simulink model "VTOL_Simulink"  (R2023a)
settings: Solver=ode4  StartTime=0.0  StopTime=100  FixedStep=0.001  RelTol=1e-3
values from neighbouring files (symbols this model uses):
  C_p = K_T/(0.5*rho*S_p*(R_p)^2)    (= 0.0365795108738)    [vtol_script.m]
  c_w = 0.35    [vtol_script.m]
  CD_0 = 0.028225    [vtol_script.m]
  CL_0 = 0.669072    [vtol_script.m]
  CL_a = 0.0904/D2R    (= 5.17953846798)    [vtol_script.m]
  Cl_beta = del_Cl_beta    (= 0.0002)    [vtol_script.m]
  Cm_0 = 0.051262    [vtol_script.m]
  Cm_a = -0.0144155/D2R    (= -0.825947309571)    [vtol_script.m]
  g = 9.8    [vtol_script.m]
  guidance_mode_on = 1    [vtol_script.m]
  K_motor = 942.3726    [vtol_script.m]
  Kinduce = 1/(pi*e*AR)    (= 0.0461549334966)    [vtol_script.m]
  m_plane = 7    [vtol_script.m]
  q_motor = 283    [vtol_script.m]
  R_p = 0.3556/2    (= 0.1778)    [vtol_script.m]
  S_p = pi*(R_p)^2    (= 0.0993146659031)    [vtol_script.m]
  S_ref = 0.704    [vtol_script.m]
  Wspan = 2.5    [vtol_script.m]
undefined symbols (not defined in the file or in its folder): alpha_thoff, Earth, sigbuilder_block, WGS84
libraries: slpidlib x13, matrix_library x4, simulink_extras x3, sharedtransform x2, aerolibasang x1, aerolibatmos2 x1, aerolibtransform2 x1, shared6dof x1
(part 2 of 2)

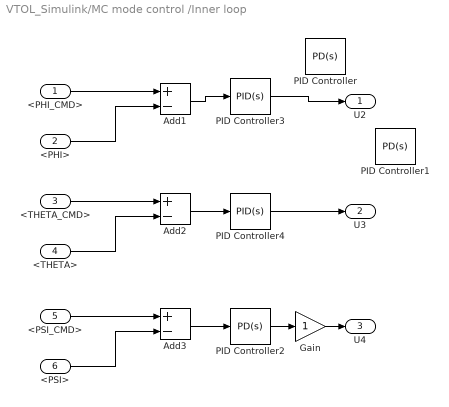
== system VTOL_Simulink/MC mode control /Inner loop ==
  " <PHI_CMD>" : Inport
  <PHI> : Inport  Port=2
  " <THETA_CMD>" : Inport  Port=3
  <THETA> : Inport  Port=4
  <PSI_CMD> : Inport  Port=5
  <PSI> : Inport  Port=6
  Add1 : Sum  Inputs=+-
  Add2 : Sum  Inputs=+-
  Add3 : Sum  Inputs=+-
  Gain : Gain
  PID Controller : slpidlib/PID Controller  Controller=PD  Form=Parallel  TimeDomain=Continuous-time  UseExternalTs=off  SampleTime=-1  IntegratorMethod=Forward Euler  FilterMethod=Forward Euler  ControllerParametersSource=internal  P=5  I=1  UseKiTs=off  D=0.5  N=100  UseFilter=on  TunerSelectOption=Transfer Function Based (PID Tuner App)  InitialConditionSource=internal  InitialConditionForIntegrator=0  InitialConditionForFilter=0  DifferentiatorICPrevScaledInput=0  ExternalReset=none  TrackingMode=off  Kt=1  LimitOutput=off  SatLimitsSource=internal  UpperSaturationLimit=inf  LowerSaturationLimit=-inf  LinearizeAsGain=on  AntiWindupMode=none  Kb=1  LimitIntegrator=off  UpperIntegratorSaturationLimit=inf  LowerIntegratorSaturationLimit=-inf  POutMin=[]  POutMax=[]  IOutMin=[]  IOutMax=[]  DOutMin=[]  DOutMax=[]  NOutMin=[]  NOutMax=[]  SumOutMin=[]  SumOutMax=[]  SaturationOutMin=[]  SaturationOutMax=[]  PParamMin=[]  PParamMax=[]  IParamMin=[]  IParamMax=[]  DParamMin=[]  DParamMax=[]  NParamMin=[]  NParamMax=[]  KbParamMin=[]  KbParamMax=[]  KtParamMin=[]  KtParamMax=[]  KbOutMin=[]  KbOutMax=[]  KtOutMin=[]  KtOutMax=[]  IntegratorOutMin=[]  IntegratorOutMax=[]  FilterOutMin=[]  FilterOutMax=[]  SumI1OutMin=[]  SumI1OutMax=[]  SumI2OutMin=[]  SumI2OutMax=[]  SumI3OutMin=[]  SumI3OutMax=[]  SumI4OutMin=[]  SumI4OutMax=[]  SumDOutMin=[]  SumDOutMax=[]  DifferentiatorOutMin=[]  DifferentiatorOutMax=[]  FilterDiffOutCoefMin=[]  FilterDiffOutCoefMax=[]  ReciprocalOutMin=[]  ReciprocalOutMax=[]  SumDenOutMin=[]  SumDenOutMax=[]  SumNumOutMin=[]  SumNumOutMax=[]  DivideOutMin=[]  DivideOutMax=[]  UdiffTsProdOutMin=[]  UdiffTsProdOutMax=[]  NTsProdOutMin=[]  NTsProdOutMax=[]  UintegralTsProdOutMin=[]  UintegralTsProdOutMax=[]  UngainTsProdOutMin=[]  UngainTsProdOutMax=[]  ClampingZeroOutDataTypeStr=Inherit: Inherit via back propagation  ClampingZeroOutMin=[]  ClampingZeroOutMax=[]  FilterDenConstantOutDataTypeStr=Inherit: Inherit via back propagation  FilterDenConstantOutMin=[]  FilterDenConstantOutMax=[]  PCopyOutDataTypeStr=Inherit: Inherit via back propagation  PCopyOutMin=[]  PCopyOutMax=[]  NCopyOutDataTypeStr=Inherit: Inherit via back propagation  NCopyOutMin=[]  NCopyOutMax=[]  IntegratorContinuousStateAttributes=''  IntegratorStateMustResolveToSignalObject=off  IntegratorRTWStateStorageClass=Auto  FilterContinuousStateAttributes=''  FilterStateMustResolveToSignalObject=off  FilterRTWStateStorageClass=Auto  ParallelPVariant=InternalParameters  IdealPVariant=Disabled  IVariant=Disabled  DVariant=InternalParameters  IntegratorVariant=Disabled  SatVariant=Disabled  AWVariant=Disabled  PCopyVariant=Disabled  TRVariant=Disabled  FdbkBlocksVariant=Forward  IdealPFdbkVariant=Disabled  SatFdbkVariant=Disabled  DerivativeFilterVariant=ContFilter  NVariant=InternalParameters  NCopyVariant=Disabled  FilterICVariant=InternalICsFilter  IntegratorICVariant=Disabled  ExternalResetVariant=Disabled  TRSumVariant=Passthrough  SumFdbkVariant=Disabled  SumVariant=Sum_PD  TsampFilterVariant=InternalTs  TsampNgainVariant=Passthrough  TsampIntegralVariant=Disabled_SignalSpec  ExternalSaturationOutDataTypeStr=Inherit: Same as second input
  PID Controller1 : slpidlib/PID Controller  Controller=PD  Form=Parallel  TimeDomain=Continuous-time  UseExternalTs=off  SampleTime=-1  IntegratorMethod=Forward Euler  FilterMethod=Forward Euler  ControllerParametersSource=internal  P=5  I=1  UseKiTs=off  D=0.5  N=100  UseFilter=on  TunerSelectOption=Transfer Function Based (PID Tuner App)  InitialConditionSource=internal  InitialConditionForIntegrator=0  InitialConditionForFilter=0  DifferentiatorICPrevScaledInput=0  ExternalReset=none  TrackingMode=off  Kt=1  LimitOutput=off  SatLimitsSource=internal  UpperSaturationLimit=inf  LowerSaturationLimit=-inf  LinearizeAsGain=on  AntiWindupMode=none  Kb=1  LimitIntegrator=off  UpperIntegratorSaturationLimit=inf  LowerIntegratorSaturationLimit=-inf  POutMin=[]  POutMax=[]  IOutMin=[]  IOutMax=[]  DOutMin=[]  DOutMax=[]  NOutMin=[]  NOutMax=[]  SumOutMin=[]  SumOutMax=[]  SaturationOutMin=[]  SaturationOutMax=[]  PParamMin=[]  PParamMax=[]  IParamMin=[]  IParamMax=[]  DParamMin=[]  DParamMax=[]  NParamMin=[]  NParamMax=[]  KbParamMin=[]  KbParamMax=[]  KtParamMin=[]  KtParamMax=[]  KbOutMin=[]  KbOutMax=[]  KtOutMin=[]  KtOutMax=[]  IntegratorOutMin=[]  IntegratorOutMax=[]  FilterOutMin=[]  FilterOutMax=[]  SumI1OutMin=[]  SumI1OutMax=[]  SumI2OutMin=[]  SumI2OutMax=[]  SumI3OutMin=[]  SumI3OutMax=[]  SumI4OutMin=[]  SumI4OutMax=[]  SumDOutMin=[]  SumDOutMax=[]  DifferentiatorOutMin=[]  DifferentiatorOutMax=[]  FilterDiffOutCoefMin=[]  FilterDiffOutCoefMax=[]  ReciprocalOutMin=[]  ReciprocalOutMax=[]  SumDenOutMin=[]  SumDenOutMax=[]  SumNumOutMin=[]  SumNumOutMax=[]  DivideOutMin=[]  DivideOutMax=[]  UdiffTsProdOutMin=[]  UdiffTsProdOutMax=[]  NTsProdOutMin=[]  NTsProdOutMax=[]  UintegralTsProdOutMin=[]  UintegralTsProdOutMax=[]  UngainTsProdOutMin=[]  UngainTsProdOutMax=[]  ClampingZeroOutDataTypeStr=Inherit: Inherit via back propagation  ClampingZeroOutMin=[]  ClampingZeroOutMax=[]  FilterDenConstantOutDataTypeStr=Inherit: Inherit via back propagation  FilterDenConstantOutMin=[]  FilterDenConstantOutMax=[]  PCopyOutDataTypeStr=Inherit: Inherit via back propagation  PCopyOutMin=[]  PCopyOutMax=[]  NCopyOutDataTypeStr=Inherit: Inherit via back propagation  NCopyOutMin=[]  NCopyOutMax=[]  IntegratorContinuousStateAttributes=''  IntegratorStateMustResolveToSignalObject=off  IntegratorRTWStateStorageClass=Auto  FilterContinuousStateAttributes=''  FilterStateMustResolveToSignalObject=off  FilterRTWStateStorageClass=Auto  ParallelPVariant=InternalParameters  IdealPVariant=Disabled  IVariant=Disabled  DVariant=InternalParameters  IntegratorVariant=Disabled  SatVariant=Disabled  AWVariant=Disabled  PCopyVariant=Disabled  TRVariant=Disabled  FdbkBlocksVariant=Forward  IdealPFdbkVariant=Disabled  SatFdbkVariant=Disabled  DerivativeFilterVariant=ContFilter  NVariant=InternalParameters  NCopyVariant=Disabled  FilterICVariant=InternalICsFilter  IntegratorICVariant=Disabled  ExternalResetVariant=Disabled  TRSumVariant=Passthrough  SumFdbkVariant=Disabled  SumVariant=Sum_PD  TsampFilterVariant=InternalTs  TsampNgainVariant=Passthrough  TsampIntegralVariant=Disabled_SignalSpec  ExternalSaturationOutDataTypeStr=Inherit: Same as second input
  PID Controller2 : slpidlib/PID Controller  Controller=PD  Form=Parallel  TimeDomain=Continuous-time  UseExternalTs=off  SampleTime=-1  IntegratorMethod=Forward Euler  FilterMethod=Forward Euler  ControllerParametersSource=internal  P=1  I=1  UseKiTs=off  D=0  N=100  UseFilter=on  TunerSelectOption=Transfer Function Based (PID Tuner App)  InitialConditionSource=internal  InitialConditionForIntegrator=0  InitialConditionForFilter=0  DifferentiatorICPrevScaledInput=0  ExternalReset=none  TrackingMode=off  Kt=1  LimitOutput=off  SatLimitsSource=internal  UpperSaturationLimit=inf  LowerSaturationLimit=-inf  LinearizeAsGain=on  AntiWindupMode=none  Kb=1  LimitIntegrator=off  UpperIntegratorSaturationLimit=inf  LowerIntegratorSaturationLimit=-inf  POutMin=[]  POutMax=[]  IOutMin=[]  IOutMax=[]  DOutMin=[]  DOutMax=[]  NOutMin=[]  NOutMax=[]  SumOutMin=[]  SumOutMax=[]  SaturationOutMin=[]  SaturationOutMax=[]  PParamMin=[]  PParamMax=[]  IParamMin=[]  IParamMax=[]  DParamMin=[]  DParamMax=[]  NParamMin=[]  NParamMax=[]  KbParamMin=[]  KbParamMax=[]  KtParamMin=[]  KtParamMax=[]  KbOutMin=[]  KbOutMax=[]  KtOutMin=[]  KtOutMax=[]  IntegratorOutMin=[]  IntegratorOutMax=[]  FilterOutMin=[]  FilterOutMax=[]  SumI1OutMin=[]  SumI1OutMax=[]  SumI2OutMin=[]  SumI2OutMax=[]  SumI3OutMin=[]  SumI3OutMax=[]  SumI4OutMin=[]  SumI4OutMax=[]  SumDOutMin=[]  SumDOutMax=[]  DifferentiatorOutMin=[]  DifferentiatorOutMax=[]  FilterDiffOutCoefMin=[]  FilterDiffOutCoefMax=[]  ReciprocalOutMin=[]  ReciprocalOutMax=[]  SumDenOutMin=[]  SumDenOutMax=[]  SumNumOutMin=[]  SumNumOutMax=[]  DivideOutMin=[]  DivideOutMax=[]  UdiffTsProdOutMin=[]  UdiffTsProdOutMax=[]  NTsProdOutMin=[]  NTsProdOutMax=[]  UintegralTsProdOutMin=[]  UintegralTsProdOutMax=[]  UngainTsProdOutMin=[]  UngainTsProdOutMax=[]  ClampingZeroOutDataTypeStr=Inherit: Inherit via back propagation  ClampingZeroOutMin=[]  ClampingZeroOutMax=[]  FilterDenConstantOutDataTypeStr=Inherit: Inherit via back propagation  FilterDenConstantOutMin=[]  FilterDenConstantOutMax=[]  PCopyOutDataTypeStr=Inherit: Inherit via back propagation  PCopyOutMin=[]  PCopyOutMax=[]  NCopyOutDataTypeStr=Inherit: Inherit via back propagation  NCopyOutMin=[]  NCopyOutMax=[]  IntegratorContinuousStateAttributes=''  IntegratorStateMustResolveToSignalObject=off  IntegratorRTWStateStorageClass=Auto  FilterContinuousStateAttributes=''  FilterStateMustResolveToSignalObject=off  FilterRTWStateStorageClass=Auto  ParallelPVariant=InternalParameters  IdealPVariant=Disabled  IVariant=Disabled  DVariant=InternalParameters  IntegratorVariant=Disabled  SatVariant=Disabled  AWVariant=Disabled  PCopyVariant=Disabled  TRVariant=Disabled  FdbkBlocksVariant=Forward  IdealPFdbkVariant=Disabled  SatFdbkVariant=Disabled  DerivativeFilterVariant=ContFilter  NVariant=InternalParameters  NCopyVariant=Disabled  FilterICVariant=InternalICsFilter  IntegratorICVariant=Disabled  ExternalResetVariant=Disabled  TRSumVariant=Passthrough  SumFdbkVariant=Disabled  SumVariant=Sum_PD  TsampFilterVariant=InternalTs  TsampNgainVariant=Passthrough  TsampIntegralVariant=Disabled_SignalSpec  ExternalSaturationOutDataTypeStr=Inherit: Same as second input
  PID Controller3 : slpidlib/PID Controller  Controller=PID  Form=Parallel  TimeDomain=Continuous-time  UseExternalTs=off  SampleTime=-1  IntegratorMethod=Forward Euler  FilterMethod=Forward Euler  ControllerParametersSource=internal  P=25  I=0.01  UseKiTs=off  D=0.01  N=100  UseFilter=on  TunerSelectOption=Transfer Function Based (PID Tuner App)  InitialConditionSource=internal  InitialConditionForIntegrator=0  InitialConditionForFilter=0  DifferentiatorICPrevScaledInput=0  ExternalReset=none  TrackingMode=off  Kt=1  LimitOutput=off  SatLimitsSource=internal  UpperSaturationLimit=inf  LowerSaturationLimit=-inf  LinearizeAsGain=on  AntiWindupMode=none  Kb=1  LimitIntegrator=off  UpperIntegratorSaturationLimit=inf  LowerIntegratorSaturationLimit=-inf  POutMin=[]  POutMax=[]  IOutMin=[]  IOutMax=[]  DOutMin=[]  DOutMax=[]  NOutMin=[]  NOutMax=[]  SumOutMin=[]  SumOutMax=[]  SaturationOutMin=[]  SaturationOutMax=[]  PParamMin=[]  PParamMax=[]  IParamMin=[]  IParamMax=[]  DParamMin=[]  DParamMax=[]  NParamMin=[]  NParamMax=[]  KbParamMin=[]  KbParamMax=[]  KtParamMin=[]  KtParamMax=[]  KbOutMin=[]  KbOutMax=[]  KtOutMin=[]  KtOutMax=[]  IntegratorOutMin=[]  IntegratorOutMax=[]  FilterOutMin=[]  FilterOutMax=[]  SumI1OutMin=[]  SumI1OutMax=[]  SumI2OutMin=[]  SumI2OutMax=[]  SumI3OutMin=[]  SumI3OutMax=[]  SumI4OutMin=[]  SumI4OutMax=[]  SumDOutMin=[]  SumDOutMax=[]  DifferentiatorOutMin=[]  DifferentiatorOutMax=[]  FilterDiffOutCoefMin=[]  FilterDiffOutCoefMax=[]  ReciprocalOutMin=[]  ReciprocalOutMax=[]  SumDenOutMin=[]  SumDenOutMax=[]  SumNumOutMin=[]  SumNumOutMax=[]  DivideOutMin=[]  DivideOutMax=[]  UdiffTsProdOutMin=[]  UdiffTsProdOutMax=[]  NTsProdOutMin=[]  NTsProdOutMax=[]  UintegralTsProdOutMin=[]  UintegralTsProdOutMax=[]  UngainTsProdOutMin=[]  UngainTsProdOutMax=[]  ClampingZeroOutDataTypeStr=Inherit: Inherit via back propagation  ClampingZeroOutMin=[]  ClampingZeroOutMax=[]  FilterDenConstantOutDataTypeStr=Inherit: Inherit via back propagation  FilterDenConstantOutMin=[]  FilterDenConstantOutMax=[]  PCopyOutDataTypeStr=Inherit: Inherit via back propagation  PCopyOutMin=[]  PCopyOutMax=[]  NCopyOutDataTypeStr=Inherit: Inherit via back propagation  NCopyOutMin=[]  NCopyOutMax=[]  IntegratorContinuousStateAttributes=''  IntegratorStateMustResolveToSignalObject=off  IntegratorRTWStateStorageClass=Auto  FilterContinuousStateAttributes=''  FilterStateMustResolveToSignalObject=off  FilterRTWStateStorageClass=Auto  ParallelPVariant=InternalParameters  IdealPVariant=Disabled  IVariant=InternalParameters  DVariant=InternalParameters  IntegratorVariant=Continuous  SatVariant=Disabled  AWVariant=Passthrough  PCopyVariant=Disabled  TRVariant=Disabled  FdbkBlocksVariant=Forward  IdealPFdbkVariant=Disabled  SatFdbkVariant=Disabled  DerivativeFilterVariant=ContFilter  NVariant=InternalParameters  NCopyVariant=Disabled  FilterICVariant=InternalICsFilter  IntegratorICVariant=InternalICs  ExternalResetVariant=Disabled  TRSumVariant=Passthrough  SumFdbkVariant=Disabled  SumVariant=Sum_PID  TsampFilterVariant=InternalTs  TsampNgainVariant=Passthrough  TsampIntegralVariant=Disabled_SignalSpec  ExternalSaturationOutDataTypeStr=Inherit: Same as second input
  PID Controller4 : slpidlib/PID Controller  Controller=PID  Form=Parallel  TimeDomain=Continuous-time  UseExternalTs=off  SampleTime=-1  IntegratorMethod=Forward Euler  FilterMethod=Forward Euler  ControllerParametersSource=internal  P=30  I=0.01  UseKiTs=off  D=0.01  N=100  UseFilter=on  TunerSelectOption=Transfer Function Based (PID Tuner App)  InitialConditionSource=internal  InitialConditionForIntegrator=0  InitialConditionForFilter=0  DifferentiatorICPrevScaledInput=0  ExternalReset=none  TrackingMode=off  Kt=1  LimitOutput=off  SatLimitsSource=internal  UpperSaturationLimit=inf  LowerSaturationLimit=-inf  LinearizeAsGain=on  AntiWindupMode=none  Kb=1  LimitIntegrator=off  UpperIntegratorSaturationLimit=inf  LowerIntegratorSaturationLimit=-inf  POutMin=[]  POutMax=[]  IOutMin=[]  IOutMax=[]  DOutMin=[]  DOutMax=[]  NOutMin=[]  NOutMax=[]  SumOutMin=[]  SumOutMax=[]  SaturationOutMin=[]  SaturationOutMax=[]  PParamMin=[]  PParamMax=[]  IParamMin=[]  IParamMax=[]  DParamMin=[]  DParamMax=[]  NParamMin=[]  NParamMax=[]  KbParamMin=[]  KbParamMax=[]  KtParamMin=[]  KtParamMax=[]  KbOutMin=[]  KbOutMax=[]  KtOutMin=[]  KtOutMax=[]  IntegratorOutMin=[]  IntegratorOutMax=[]  FilterOutMin=[]  FilterOutMax=[]  SumI1OutMin=[]  SumI1OutMax=[]  SumI2OutMin=[]  SumI2OutMax=[]  SumI3OutMin=[]  SumI3OutMax=[]  SumI4OutMin=[]  SumI4OutMax=[]  SumDOutMin=[]  SumDOutMax=[]  DifferentiatorOutMin=[]  DifferentiatorOutMax=[]  FilterDiffOutCoefMin=[]  FilterDiffOutCoefMax=[]  ReciprocalOutMin=[]  ReciprocalOutMax=[]  SumDenOutMin=[]  SumDenOutMax=[]  SumNumOutMin=[]  SumNumOutMax=[]  DivideOutMin=[]  DivideOutMax=[]  UdiffTsProdOutMin=[]  UdiffTsProdOutMax=[]  NTsProdOutMin=[]  NTsProdOutMax=[]  UintegralTsProdOutMin=[]  UintegralTsProdOutMax=[]  UngainTsProdOutMin=[]  UngainTsProdOutMax=[]  ClampingZeroOutDataTypeStr=Inherit: Inherit via back propagation  ClampingZeroOutMin=[]  ClampingZeroOutMax=[]  FilterDenConstantOutDataTypeStr=Inherit: Inherit via back propagation  FilterDenConstantOutMin=[]  FilterDenConstantOutMax=[]  PCopyOutDataTypeStr=Inherit: Inherit via back propagation  PCopyOutMin=[]  PCopyOutMax=[]  NCopyOutDataTypeStr=Inherit: Inherit via back propagation  NCopyOutMin=[]  NCopyOutMax=[]  IntegratorContinuousStateAttributes=''  IntegratorStateMustResolveToSignalObject=off  IntegratorRTWStateStorageClass=Auto  FilterContinuousStateAttributes=''  FilterStateMustResolveToSignalObject=off  FilterRTWStateStorageClass=Auto  ParallelPVariant=InternalParameters  IdealPVariant=Disabled  IVariant=InternalParameters  DVariant=InternalParameters  IntegratorVariant=Continuous  SatVariant=Disabled  AWVariant=Passthrough  PCopyVariant=Disabled  TRVariant=Disabled  FdbkBlocksVariant=Forward  IdealPFdbkVariant=Disabled  SatFdbkVariant=Disabled  DerivativeFilterVariant=ContFilter  NVariant=InternalParameters  NCopyVariant=Disabled  FilterICVariant=InternalICsFilter  IntegratorICVariant=InternalICs  ExternalResetVariant=Disabled  TRSumVariant=Passthrough  SumFdbkVariant=Disabled  SumVariant=Sum_PID  TsampFilterVariant=InternalTs  TsampNgainVariant=Passthrough  TsampIntegralVariant=Disabled_SignalSpec  ExternalSaturationOutDataTypeStr=Inherit: Same as second input
  " U2" : Outport
  U3 : Outport  Port=2
  U4 : Outport  Port=3
  wires:
  <PHI>/1 -> Add1/2
  <THETA>/1 -> Add2/2
  <PSI>/1 -> Add3/2
  Add1/1 -> PID Controller3/1
  Add2/1 -> PID Controller4/1
  Add3/1 -> PID Controller2/1
  PID Controller3/1 -> " U2"/1
  PID Controller4/1 -> U3/1
  PID Controller2/1 -> Gain/1
  <PSI_CMD>/1 -> Add3/1
  Gain/1 -> U4/1
  " <PHI_CMD>"/1 -> Add1/1
  " <THETA_CMD>"/1 -> Add2/1

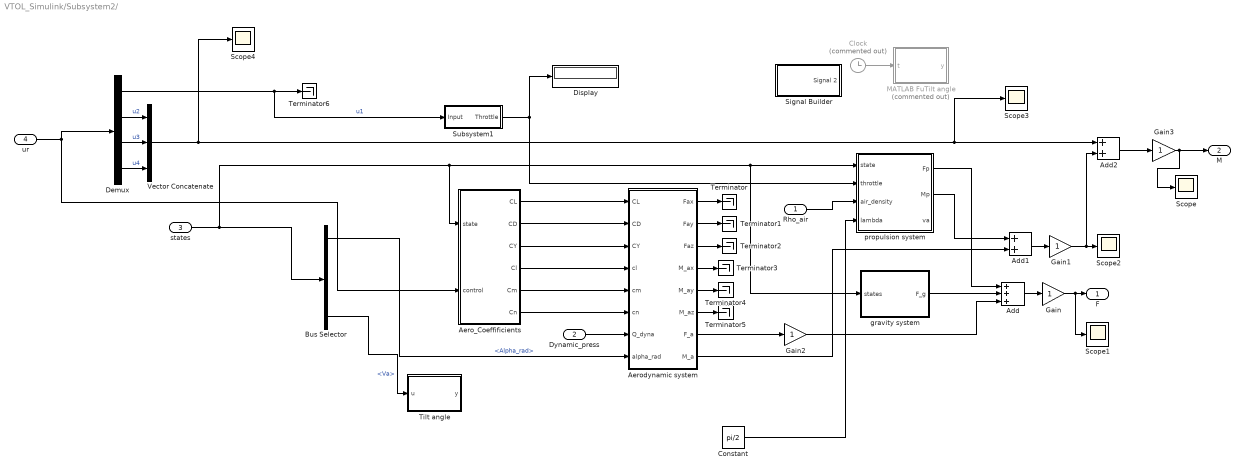
== system VTOL_Simulink/Subsystem2/  ==
  " Rho_air" : Inport
  Dynamic_press : Inport  Port=2
  states : Inport  Port=3
  ur : Inport  Port=4
  " Aero_Coeffificients" : Subsystem
  " gravity system" : Subsystem
  " propulsion system" : Subsystem
  Add : Sum  Inputs=+++
  Add1 : Sum
  Add2 : Sum
  Aerodynamic system : Subsystem
  Bus Selector : BusSelector  OutputSignals=Alpha_rad,pn pe pd,Euler_ang_rad,Va
  Clock : Clock  Commented=on
  Constant : Constant  Value=pi/2
  Demux : Demux  Outputs=04
  Display : Display
  Gain{,1..3} (4 alike) : Gain
  MATLAB FuTilt angle : MATLAB Function  Commented=on  TreatAsAtomicUnit=on
  Scope{,1..4} (5 alike) : Scope
  Signal Builder : Subsystem  Tag=STV Subsys  LoadFcn=sigbuilder_block('load');  StartFcn=sigbuilder_block('start');  StopFcn=sigbuilder_block('stop');  ClipboardFcn=sigbuilder_block('clipboard');  mask(Sigbuilder block){tuvar=[0:10]}
      mask help: Simulink:masks:SigbuilderBlock_MD
      mask init:
      | if ~strcmp(get_param(bdroot(gcbh),'SimulationStatus'),'stopped') tuvar = sigbuilder_block('maskInit'); end
      settings: CopyFcn=sigbuilder_block('copy');  DeleteFcn=sigbuilder_block('delete');  ModelCloseFcn=sigbuilder_block('modelClose');  PreSaveFcn=sigbuilder_block('preSave');  PauseFcn=sigbuilder_block('pause');  ContinueFcn=sigbuilder_block('continue');  NameChangeFcn=sigbuilder_block('namechange');  OpenFcn=sigbuilder_block('open',[5.4 36 1141.2 516.6 ]);  CloseFcn=sigbuilder_block('close');
      mask Display: plot(0, 0, 100, 100,[2, 2, 32, 32, 2], [68, 8, 8, 68, 68],[32, 2], [38, 38], [32, 19, 2],[53, 60, 44], [32, 17, 17, 2],[16, 16, 31, 31]);txt = getActiveGroup(gcbh);text(2, 100, txt,'verticalAlignment', 'top');
  Subsystem1 : Subsystem
  Terminator{,1..6} (7 alike) : Terminator
  Tilt angle : MATLAB Function  TreatAsAtomicUnit=on
  Vector Concatenate : Concatenate  NumInputs=03
  F : Outport
  " M" : Outport  Port=2
  wires:
  Aerodynamic system/4(" M_ax") -> Terminator3/1
  " Aero_Coeffificients"/4("  Cl") -> Aerodynamic system/4(" cl")
  " Aero_Coeffificients"/5("  Cm") -> Aerodynamic system/5(" cm")
  Aerodynamic system/5(M_ay) -> Terminator4/1
  Aerodynamic system/2(" Fay") -> Terminator1/1
  Add/1 -> Gain/1
  Aerodynamic system/3(" Faz") -> Terminator2/1
  " Aero_Coeffificients"/6(" Cn") -> Aerodynamic system/6(" cn")
  " Aero_Coeffificients"/1(" CL") -> Aerodynamic system/1(CL)
  Aerodynamic system/1(" Fax") -> Terminator/1
  Aerodynamic system/6(" M_az") -> Terminator5/1
  " Aero_Coeffificients"/2(" CD") -> Aerodynamic system/2(CD)
  " Aero_Coeffificients"/3(" CY") -> Aerodynamic system/3(CY)
  Dynamic_press/1 -> Aerodynamic system/7(" Q_dyna")
  Bus Selector/1 -> Aerodynamic system/8("  alpha_rad")  "<Alpha_rad>"
  " Rho_air"/1 -> " propulsion system"/3(" air_density")
  Aerodynamic system/7(" F_a") -> Gain2/1
  Aerodynamic system/8(" M_a") -> Add1/2
  " propulsion system"/2(" Mp") -> Add1/1
  Add1/1 -> Gain1/1
  states/1 -> Bus Selector/1, " Aero_Coeffificients"/1(" state"), " gravity system"/1(states), " propulsion system"/1(" state")
  Gain/1 -> Scope1/1, F/1
  Gain2/1 -> Add/3
  Clock/1 -> MATLAB FuTilt angle/1(t)
  Subsystem1/1(" Throttle") -> Display/1, " propulsion system"/2(" throttle")
  " propulsion system"/1(" Fp") -> Add/1
  " gravity system"/1(F_g) -> Add/2
  ur/1 -> " Aero_Coeffificients"/2(" control"), Demux/1
  Demux/1 -> Subsystem1/1(Input), Terminator6/1  "u1"
  Bus Selector/4 -> Tilt angle/1(u)  "<Va>"
  Vector Concatenate/1 -> Scope4/1, Scope3/1, Add2/1
  Demux/2 -> Vector Concatenate/1  "u2"
  Demux/3 -> Vector Concatenate/2  "u3"
  Demux/4 -> Vector Concatenate/3  "u4"
  Add2/1 -> Gain3/1
  Gain1/1 -> Add2/2, Scope2/1
  Gain3/1 -> Scope/1, " M"/1
  Constant/1 -> " propulsion system"/4(" lambda")

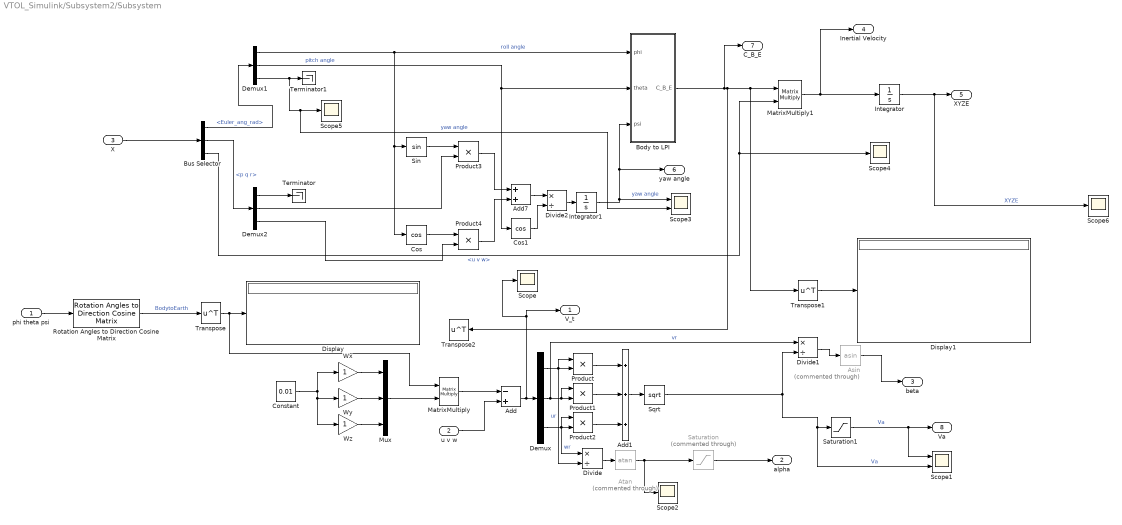
== system VTOL_Simulink/Subsystem2/Subsystem ==
  " phi theta psi" : Inport
  " u v w" : Inport  Port=2
  " X" : Inport  Port=3
  " Body to LPI" : Subsystem
  " Wx" : Gain
  Add : Sum  Inputs=-+
  Add1 : Sum  Inputs=+++
  Add7 : Sum
  Asin : Trigonometry  Commented=through  Operator=asin
  Atan : Trigonometry  Commented=through  Operator=atan
  Bus Selector : BusSelector  OutputSignals=Euler_ang_rad,p q r,u v w
  Constant : Constant  Value=0.01
  Cos : Trigonometry  Operator=cos
  Cos1 : Trigonometry  Operator=cos
  Demux : Demux  Outputs=03
  Demux1 : Demux  Outputs=03
  Demux2 : Demux  Outputs=03
  Display : Display
  Display1 : Display
  Divide : Product  Inputs=*/
  Divide1 : Product  Inputs=*/
  Divide2 : Product  Inputs=*/
  Integrator : Integrator
  Integrator1 : Integrator
  MatrixMultiply : Product  Multiplication=Matrix(*)
  MatrixMultiply1 : Product  Multiplication=Matrix(*)
  Mux : Mux  Inputs=03
  Product{,1..4} (5 alike) : Product
  Rotation Angles to Direction Cosine Matrix : sharedtransform/Rotation Angles to Direction Cosine Matrix  rotationOrder=ZYX  aMode=aMode
  Saturation : Saturate  Commented=through  UpperLimit=pi/6  LowerLimit=-pi/6
  Saturation1 : Saturate  UpperLimit=25  LowerLimit=0
  Scope{,2,4..6} (5 alike) : Scope
  Scope1 : Scope  NumInputPorts=2
  Scope3 : Scope  NumInputPorts=2
  Sin : Trigonometry
  Sqrt : Sqrt
  Terminator : Terminator
  Terminator1 : Terminator
  Transpose : Math  Operator=transpose
  Transpose1 : Math  Operator=transpose
  Transpose2 : Math  Operator=transpose
  Wy : Gain
  Wz : Gain
  " V_t" : Outport
  " alpha" : Outport  Port=2
  " beta" : Outport  Port=3
  " Inertial Velocity " : Outport  Port=4
  XYZE : Outport  Port=5
  yaw angle : Outport  Port=6
  C_B_E : Outport  Port=7
  Va : Outport  Port=8
  wires:
  " u v w"/1 -> Add/2
  " phi theta psi"/1 -> Rotation Angles to Direction Cosine Matrix/1
  Rotation Angles to Direction Cosine Matrix/1 -> Transpose/1  "BodytoEarth"
  Constant/1 -> Wz/1, Wy/1, " Wx"/1
  " Wx"/1 -> Mux/1
  Wy/1 -> Mux/2
  Wz/1 -> Mux/3
  Mux/1 -> MatrixMultiply/2
  MatrixMultiply/1 -> Add/1
  Add/1 -> Scope/1, " V_t"/1, Demux/1
  Demux/1 -> Product/2, Divide/2, Product/1  "ur"
  Demux/2 -> Product1/1, Product1/2, Divide1/1  "vr"
  Demux/3 -> Divide/1, Product2/1, Product2/2  "wr"
  Product/1 -> Add1/1
  Product1/1 -> Add1/2
  Product2/1 -> Add1/3
  Add1/1 -> Sqrt/1
  Sqrt/1 -> Scope1/2, Saturation1/1, Divide1/2  "Va"
  Divide/1 -> Atan/1
  Divide1/1 -> Asin/1
  Atan/1 -> Scope2/1, Saturation/1
  Asin/1 -> " beta"/1
  Cos/1 -> Product4/1
  Demux2/3 -> Product4/2
  Demux1/3 -> Scope3/2, Scope5/1, Terminator1/1  "yaw angle"
  Demux1/2 -> Cos1/1, " Body to LPI"/2(theta)  "pitch angle"
  Demux2/1 -> Terminator/1
  Cos1/1 -> Divide2/2
  Divide2/1 -> Integrator1/1
  Add7/1 -> Divide2/1
  MatrixMultiply1/1 -> Integrator/1, " Inertial Velocity "/1
  Product4/1 -> Add7/2
  Integrator1/1 -> Scope3/1, " Body to LPI"/3(psi), yaw angle/1  "yaw angle"
  Sin/1 -> Product3/1
  Demux2/2 -> Product3/2
  Integrator/1 -> Scope6/1, XYZE/1  "XYZE"
  Product3/1 -> Add7/1
  Demux1/1 -> Cos/1, Sin/1, " Body to LPI"/1(phi)  "roll angle"
  " X"/1 -> Bus Selector/1
  Bus Selector/1 -> Demux1/1  "<Euler_ang_rad>"
  Bus Selector/2 -> Demux2/1  "<p q r>"
  Bus Selector/3 -> MatrixMultiply1/2, Scope4/1  "<u v w>"
  " Body to LPI"/1(C_B_E) -> C_B_E/1, Transpose2/1, Transpose1/1, MatrixMultiply1/1
  Transpose/1 -> MatrixMultiply/1, Display/1
  Transpose1/1 -> Display1/1
  Saturation/1 -> " alpha"/1
  Saturation1/1 -> Scope1/1, Va/1  "Va"

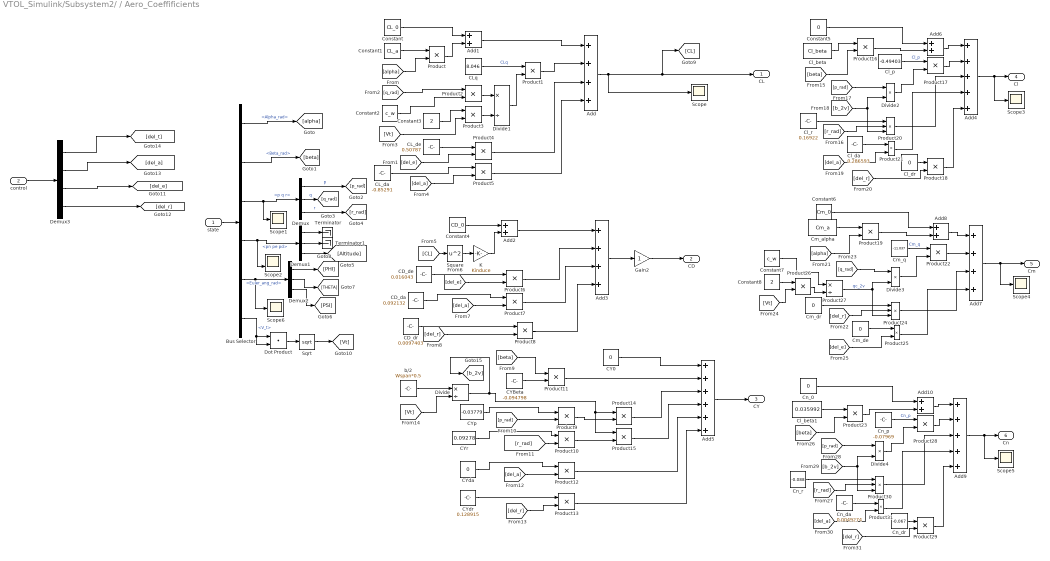
== system VTOL_Simulink/Subsystem2/ / Aero_Coeffificients ==
  " state" : Inport
  " control" : Inport  Port=2
  " CD_da" : Constant  Value=0.092132
  " CD_de" : Constant  Value=0.016043
  " CD_dr" : Constant  Value=0.0097403
  " CL_da" : Constant  Value=-0.85291
  " CL_de" : Constant  Value=0.50787
  " CLq" : Constant  Value=8.046
  " CY0" : Constant  Value=0
  " CYda" : Constant  Value=0
  " CYdr" : Constant  Value=0.128915
  " CYp" : Constant  Value=-0.03779
  " CYr" : Constant  Value=0.09278
  " Cl_beta" : Constant  Value=Cl_beta
  " Cl_beta1" : Constant  Value=0.035992
  " Cl_da" : Constant  Value=0.286593
  " Cl_dr" : Constant  Value=0
  " Cl_p" : Constant  Value=-0.49403
  " Cl_r" : Constant  Value=0.16922
  " Cm_alpha" : Constant  Value=Cm_a
  " Cm_de" : Constant  Value=0
  " Cm_dr" : Constant  Value=0
  " Cm_q" : Constant  Value=-11.037
  " Cn_0" : Constant  Value=0
  " Cn_da" : Constant  Value=0.0049274
  " Cn_dr" : Constant  Value=-0.067
  " Cn_p" : Constant  Value=-0.07969
  " Cn_r" : Constant  Value=-0.088
  " b/2" : Constant  Value=Wspan*0.5
  Add : Sum  Inputs=++++
  Add{1..2,6,8,10} (5 alike) : Sum
  Add3 : Sum  Inputs=++++
  Add4 : Sum  Inputs=+++++
  Add5 : Sum  Inputs=++++++
  Add7 : Sum  Inputs=++++
  Add9 : Sum  Inputs=+++++
  Bus Selector : BusSelector  OutputSignals=Alpha_rad,Beta_rad,p q r,pn pe pd,Euler_ang_rad,V_t
  CYBeta : Constant  Value=-0.094798
  Constant : Constant  Value=CL_0
  Constant1 : Constant  Value=CL_a
  Constant2 : Constant  Value=c_w
  Constant3 : Constant  Value=2
  Constant4 : Constant  Value=CD_0
  Constant5 : Constant  Value=0
  Constant6 : Constant  Value=Cm_0
  Constant7 : Constant  Value=c_w
  Constant8 : Constant  Value=2
  Demux : Demux  Outputs=03
  Demux1 : Demux  Outputs=03
  Demux2 : Demux  Outputs=03
  Demux3 : Demux  Outputs=04
  Divide : Product  Inputs=*/
  Divide1 : Product  Inputs=*/
  Divide2 : Product  Inputs=**
  Divide3 : Product  Inputs=**
  Divide4 : Product  Inputs=**
  Dot Product : DotProduct  OutDataTypeStr=Inherit: Inherit via internal rule
  Gain2 : Gain
  K : Gain  Gain=Kinduce
  Product{,1..19,21..23,25..26,28..29,31} (28 alike) : Product
  Product20 : Product  Inputs=3
  Product24 : Product  Inputs=3
  Product27 : Product  Inputs=*/
  Product30 : Product  Inputs=3
  Scope{,1,3..6} (6 alike) : Scope
  Scope2 : Scope  NumInputPorts=2
  Sqrt : Sqrt
  Square : Math  Operator=square
  Terminator : Terminator
  Terminator1 : Terminator
  " CL" : Outport
  " CD" : Outport  Port=2
  " CY" : Outport  Port=3
  "  Cl" : Outport  Port=4
  "  Cm" : Outport  Port=5
  " Cn" : Outport  Port=6
  wires:
  " state"/1 -> Bus Selector/1
  Bus Selector/1 -> [alpha]  "<Alpha_rad>"
  Bus Selector/2 -> [beta]  "<Beta_rad>"
  Bus Selector/3 -> Scope1/1, Demux/1  "<p q r>"
  Demux/1 -> [p_rad]  "p"
  Demux/2 -> [q_rad]  "q"
  Demux/3 -> [r_rad]  "r"
  Bus Selector/4 -> Scope2/2, Demux1/1  "<pn pe pd>"
  Bus Selector/5 -> Demux2/1, Scope6/1  "<Euler_ang_rad>"
  Demux1/1 -> Terminator/1
  Demux1/2 -> Terminator1/1
  Demux1/3 -> [Altitude]
  Demux2/3 -> [PSI]
  Demux2/2 -> [THETA]
  Demux2/1 -> [PHI]
  Constant/1 -> Add1/1
  [alpha] -> Product/2
  Constant1/1 -> Product/1
  Product/1 -> Add1/2
  Add1/1 -> Add/1
  [q_rad] -> Product2/1
  " CLq"/1 -> Product1/1  "CLq"
  Constant2/1 -> Product2/2
  Product2/1 -> Divide1/1
  Constant3/1 -> Product3/1
  [Vt] -> Product3/2
  Product3/1 -> Divide1/2
  Divide1/1 -> Product1/2
  Product1/1 -> Add/2
  " CL_de"/1 -> Product4/1
  [del_e] -> Product4/2
  " CL_da"/1 -> Product5/1
  [del_a] -> Product5/2
  Product4/1 -> Add/3
  Product5/1 -> Add/4
  Constant4/1 -> Add2/1
  [CL] -> Square/1
  Square/1 -> K/1
  K/1 -> Add2/2
  Add2/1 -> Add3/1
  [del_e] -> Product6/2
  " CD_da"/1 -> Product7/1
  Product6/1 -> Add3/2
  [del_a] -> Product7/2
  Product7/1 -> Add3/3
  " CD_de"/1 -> Product6/1
  [del_r] -> Product8/2
  " CD_dr"/1 -> Product8/1
  Product8/1 -> Add3/4
  Add3/1 -> Gain2/1
  " CYp"/1 -> Product9/1
  [r_rad] -> Product10/2
  " CYr"/1 -> Product10/1
  [p_rad] -> Product9/2
  Add5/1 -> " CY"/1
  " CY0"/1 -> Add5/1
  CYBeta/1 -> Product11/2
  [beta] -> Product11/1
  Product11/1 -> Add5/2
  " CYda"/1 -> Product12/1
  [del_a] -> Product12/2
  " CYdr"/1 -> Product13/1
  [del_r] -> Product13/2
  " b/2"/1 -> Divide/1
  [Vt] -> Divide/2
  Divide/1 -> Product15/1, Product14/1, [b_2v]
  Product9/1 -> Product14/2
  Product10/1 -> Product15/2
  Product14/1 -> Add5/3
  Product15/1 -> Add5/4
  Product12/1 -> Add5/5
  Product13/1 -> Add5/6
  Bus Selector/6 -> Dot Product/1, Dot Product/2  "<V_t>"
  Dot Product/1 -> Sqrt/1
  Sqrt/1 -> [Vt]
  " Cl_r"/1 -> Product20/1
  Add4/1 -> Scope3/1, "  Cl"/1
  " Cl_da"/1 -> Product21/1
  " Cl_beta"/1 -> Product16/1
  [r_rad] -> Product20/2
  Product16/1 -> Add6/2
  Product20/1 -> Add4/3
  [p_rad] -> Divide2/1
  Add6/1 -> Add4/1
  " Cl_p"/1 -> Product17/1  "Cl_p"
  [del_a] -> Product21/2
  Product17/1 -> Add4/2
  Constant5/1 -> Add6/1
  [beta] -> Product16/2
  Product21/1 -> Add4/4
  [b_2v] -> Product20/3, Divide2/2
  Divide2/1 -> Product17/2
  [del_r] -> Product18/2
  Product18/1 -> Add4/5
  " Cl_dr"/1 -> Product18/1
  Product27/1 -> Product24/3, Divide3/2  "qc_2v"
  Constant6/1 -> Add8/1
  [del_e] -> Product25/2
  " Cm_q"/1 -> Product22/1  "Cm_q"
  Product25/1 -> Add7/4
  " Cm_de"/1 -> Product25/1
  Product24/1 -> Add7/3
  [del_r] -> Product24/2
  " Cm_alpha"/1 -> Product19/1
  Add8/1 -> Add7/1
  " Cm_dr"/1 -> Product24/1
  Add7/1 -> Scope4/1, "  Cm"/1
  [alpha] -> Product19/2
  Product22/1 -> Add7/2
  Product19/1 -> Add8/2
  [q_rad] -> Divide3/1
  Divide3/1 -> Product22/2
  Constant8/1 -> Product26/1
  Constant7/1 -> Product27/1
  [Vt] -> Product26/2
  Product26/1 -> Product27/2
  [b_2v] -> Product30/3, Divide4/2
  " Cn_dr"/1 -> Product29/1
  " Cn_0"/1 -> Add10/1
  [del_a] -> Product31/2
  " Cn_p"/1 -> Product28/1  "Cn_p"
  Product31/1 -> Add9/4
  " Cn_da"/1 -> Product31/1
  Product30/1 -> Add9/3
  [r_rad] -> Product30/2
  " Cl_beta1"/1 -> Product23/1
  Add10/1 -> Add9/1
  " Cn_r"/1 -> Product30/1
  Add9/1 -> " Cn"/1, Scope5/1
  [beta] -> Product23/2
  Product29/1 -> Add9/5
  Product28/1 -> Add9/2
  Product23/1 -> Add10/2
  [p_rad] -> Divide4/1
  Divide4/1 -> Product28/2
  [del_r] -> Product29/2
  Gain2/1 -> " CD"/1
  Add/1 -> " CL"/1, [CL], Scope/1
  Demux3/4 -> [del_r]
  Demux3/2 -> [del_a]
  Demux3/3 -> [del_e]
  " control"/1 -> Demux3/1
  Demux3/1 -> [del_t]

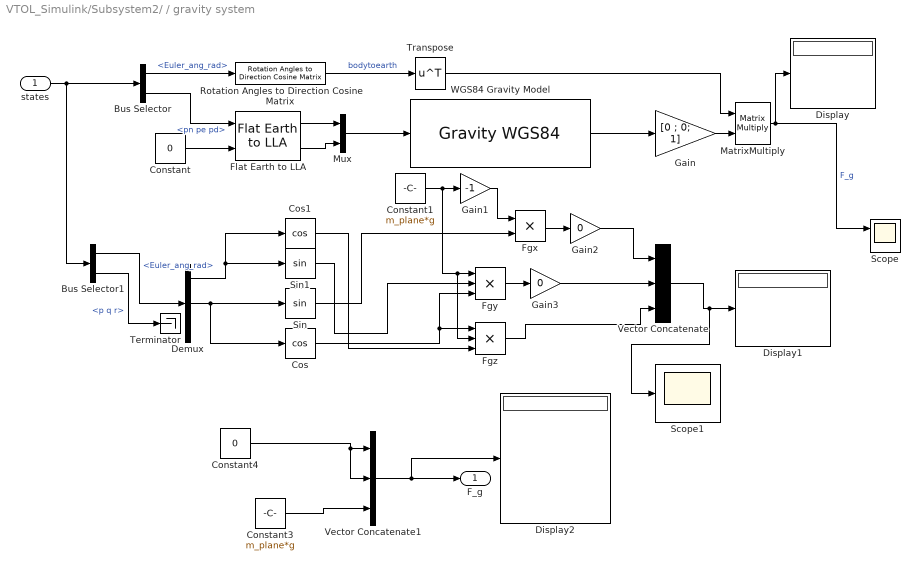
== system VTOL_Simulink/Subsystem2/ / gravity system ==
  states : Inport
  " Fgy" : Product  Inputs=3
  " Fgz" : Product  Inputs=03
  Bus Selector : BusSelector  OutputSignals=Euler_ang_rad,pn pe pd
  Bus Selector1 : BusSelector  OutputSignals=Euler_ang_rad,p q r
  Constant : Constant  Value=0
  Constant1 : Constant  Value=m_plane*g
  Constant3 : Constant  Value=m_plane*g
  Constant4 : Constant  Value=0
  Cos : Trigonometry  Operator=cos
  Cos1 : Trigonometry  Operator=cos
  Demux : Demux  Outputs=03
  Display : Display
  Display1 : Display
  Display2 : Display
  Fgx : Product
  Flat Earth to LLA : aerolibtransform2/Flat Earth to LLA  units=Metric (MKS)  ptype=Earth (WGS84)  F=1/298.257223563  R=6378137  refPosPort=off  LL0=[0 10]  psi=0
  Gain : Gain  Gain=[0 ; 0; 1]
  Gain1 : Gain  Gain=-1
  Gain2 : Gain  Gain=0
  Gain3 : Gain  Gain=0
  MatrixMultiply : Product  Multiplication=Matrix(*)
  Mux : Mux  Inputs=2
  Rotation Angles to Direction Cosine Matrix : sharedtransform/Rotation Angles to Direction Cosine Matrix  rotationOrder=ZYX  aMode=aMode
  Scope : Scope  NumInputPorts=2
  Scope1 : Scope
  Sin : Trigonometry
  Sin1 : Trigonometry
  Terminator : Terminator
  Transpose : Math  Operator=transpose
  Vector Concatenate : Concatenate  NumInputs=03
  Vector Concatenate1 : Concatenate  NumInputs=03
  "WGS84 Gravity Model  " : GravityWGS84
  F_g : Outport
  wires:
  states/1 -> Bus Selector1/1, Bus Selector/1
  Flat Earth to LLA/2 -> Mux/2
  Bus Selector/1 -> Rotation Angles to Direction Cosine Matrix/1  "<Euler_ang_rad>"
  Constant/1 -> Flat Earth to LLA/2
  Mux/1 -> "WGS84 Gravity Model  "/1
  "WGS84 Gravity Model  "/1 -> Gain/1
  Gain/1 -> MatrixMultiply/2
  Rotation Angles to Direction Cosine Matrix/1 -> Transpose/1  "bodytoearth"
  Flat Earth to LLA/1 -> Mux/1
  Bus Selector/2 -> Flat Earth to LLA/1  "<pn pe pd>"
  Transpose/1 -> MatrixMultiply/1
  MatrixMultiply/1 -> Scope/1, Display/1  "F_g"
  Bus Selector1/1 -> Demux/1  "<Euler_ang_rad>"
  Bus Selector1/2 -> Terminator/1  "<p q r>"
  Demux/2 -> Cos/1, Sin/1
  Demux/1 -> Cos1/1, Sin1/1
  Sin/1 -> Fgx/2
  Cos/1 -> " Fgy"/3, " Fgz"/1
  Sin1/1 -> " Fgy"/2
  Cos1/1 -> " Fgz"/3
  Constant1/1 -> " Fgz"/2, " Fgy"/1, Gain1/1
  Gain1/1 -> Fgx/1
  Fgx/1 -> Gain2/1
  " Fgy"/1 -> Gain3/1
  " Fgz"/1 -> Vector Concatenate/3
  Vector Concatenate/1 -> Scope1/1, Display1/1
  Gain3/1 -> Vector Concatenate/2
  Gain2/1 -> Vector Concatenate/1
  Constant3/1 -> Vector Concatenate1/3
  Constant4/1 -> Vector Concatenate1/2, Vector Concatenate1/1
  Vector Concatenate1/1 -> Display2/1, F_g/1

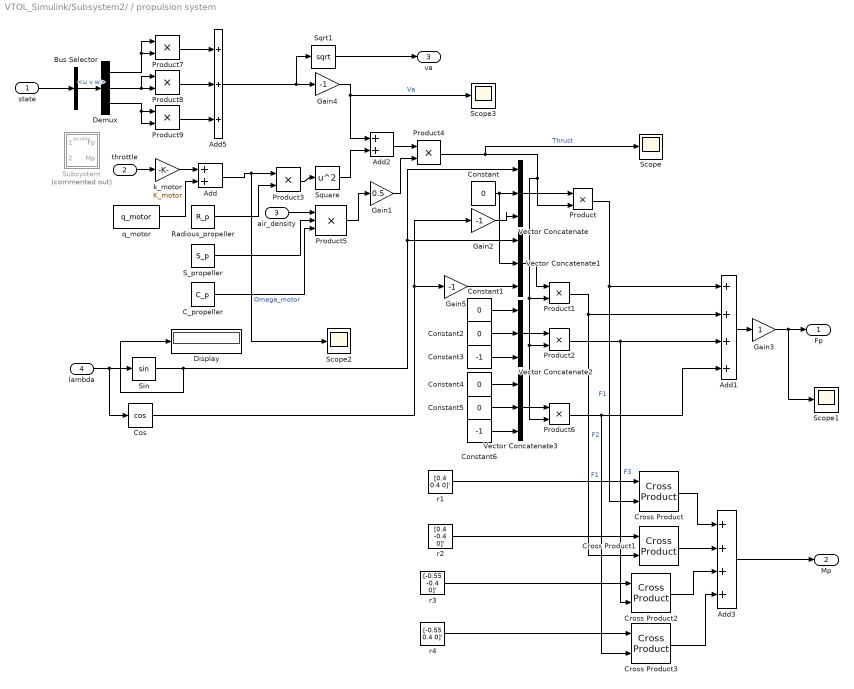
== system VTOL_Simulink/Subsystem2/ / propulsion system ==
  " state" : Inport
  " throttle" : Inport  Port=2
  " air_density" : Inport  Port=3
  " lambda" : Inport  Port=4
  "  r1" : Constant  Value="[0.4  0.4  0]'"
  "  r2" : Constant  Value="[0.4  -0.4  0]'"
  "  r3" : Constant  Value="[-0.55 -0.4  0]'"
  "  r4" : Constant  Value="[-0.55  0.4 0]'"
  " C_propeller" : Constant  Value=C_p
  " Radious_propeller" : Constant  Value=R_p
  " S_propeller" : Constant  Value=S_p
  " k_motor" : Gain  Gain=K_motor
  " q_motor" : Constant  Value=q_motor
  Add : Sum
  Add1 : Sum  Inputs=++++
  Add2 : Sum
  Add3 : Sum  Inputs=++++
  Add5 : Sum  Inputs=+++
  Bus Selector : BusSelector  OutputSignals=u v w
  Constant{,1..2,4..5} (5 alike) : Constant  Value=0
  Constant3 : Constant  Value=-1
  Constant6 : Constant  Value=-1
  Cos : Trigonometry  Operator=cos
  Cross Product{,1..3} (4 alike) : matrix_library/Cross Product
  Demux : Demux  Outputs=03
  Display : Display
  Gain1 : Gain  Gain=0.5
  Gain2 : Gain  Gain=-1
  Gain3 : Gain
  Gain4 : Gain  Gain=-1
  Gain5 : Gain  Gain=-1
  Product{,1..4,6..9} (9 alike) : Product
  Product5 : Product  Inputs=03
  Scope{,1..3} (4 alike) : Scope
  Sin : Trigonometry
  Sqrt1 : Sqrt
  Square : Math  Operator=square
  Subsystem : Subsystem  Commented=on
  Vector Concatenate{,1..3} (4 alike) : Concatenate  NumInputs=03
  " Fp" : Outport
  " Mp" : Outport  Port=2
  " va" : Outport  Port=3
  wires:
  " state"/1 -> Bus Selector/1
  " throttle"/1 -> " k_motor"/1
  " k_motor"/1 -> Add/1
  " q_motor"/1 -> Add/2
  Add/1 -> Scope2/1, Product3/1  "Omega_motor"
  " Radious_propeller"/1 -> Product3/2
  Product3/1 -> Square/1
  Square/1 -> Add2/2
  Add2/1 -> Product4/1
  " air_density"/1 -> Product5/1
  " S_propeller"/1 -> Product5/2
  " C_propeller"/1 -> Product5/3
  Product5/1 -> Gain1/1
  Gain1/1 -> Product4/2
  " lambda"/1 -> Cos/1, Sin/1
  Vector Concatenate/1 -> Product/1
  Product4/1 -> Scope/1, Product6/2, Product2/2, Product1/2, Product/2  "Thrust"
  Vector Concatenate1/1 -> Product1/1
  Vector Concatenate2/1 -> Product2/1
  Vector Concatenate3/1 -> Product6/1
  Sin/1 -> Display/1, Vector Concatenate/1, Vector Concatenate1/1
  Constant/1 -> Vector Concatenate1/2, Vector Concatenate/2
  Cos/1 -> Gain2/1, Gain5/1
  Gain2/1 -> Vector Concatenate/3
  Constant3/1 -> Vector Concatenate2/3
  Constant2/1 -> Vector Concatenate2/2
  Constant1/1 -> Vector Concatenate2/1
  Constant4/1 -> Vector Concatenate3/1
  Constant5/1 -> Vector Concatenate3/2
  Constant6/1 -> Vector Concatenate3/3
  Product1/1 -> Cross Product1/2, Add1/2  "F2"
  Add1/1 -> Gain3/1
  "  r1"/1 -> Cross Product/1
  Product/1 -> Cross Product/2, Add1/1  "F1"
  "  r2"/1 -> Cross Product1/1
  Product2/1 -> Cross Product2/2, Add1/3  "F3"
  "  r3"/1 -> Cross Product2/1
  Product6/1 -> Cross Product3/2, Add1/4  "F1"
  "  r4"/1 -> Cross Product3/1
  Cross Product/1 -> Add3/1
  Cross Product1/1 -> Add3/2
  Cross Product2/1 -> Add3/3
  Cross Product3/1 -> Add3/4
  Add3/1 -> " Mp"/1
  Gain3/1 -> Scope1/1, " Fp"/1
  Gain4/1 -> Add2/1, Scope3/1  "Va"
  Demux/2 -> Product8/1, Product8/2
  Product9/1 -> Add5/3
  Demux/3 -> Product9/2, Product9/1
  Product8/1 -> Add5/2
  Demux/1 -> Product7/1, Product7/2
  Product7/1 -> Add5/1
  Bus Selector/1 -> Demux/1  "<u v w>"
  Gain5/1 -> Vector Concatenate1/3
  Add5/1 -> Sqrt1/1, Gain4/1
  Sqrt1/1 -> " va"/1

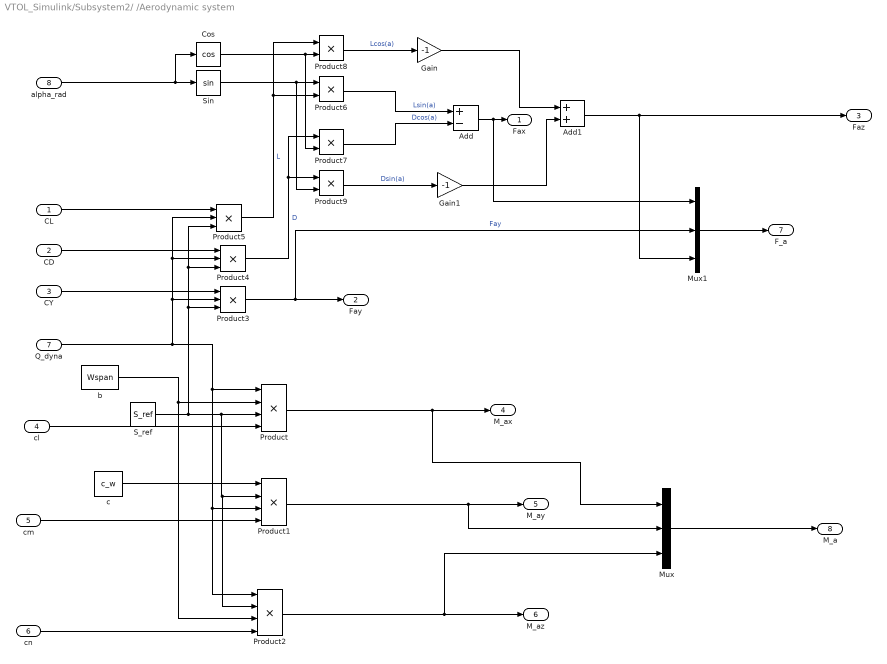
== system VTOL_Simulink/Subsystem2/ /Aerodynamic system ==
  CL : Inport
  CD : Inport  Port=2
  CY : Inport  Port=3
  " cl" : Inport  Port=4
  " cm" : Inport  Port=5
  " cn" : Inport  Port=6
  " Q_dyna" : Inport  Port=7
  "  alpha_rad" : Inport  Port=8
  "  S_ref" : Constant  Value=S_ref
  " b" : Constant  Value=Wspan
  " c" : Constant  Value=c_w
  Add : Sum  Inputs=+-
  Add1 : Sum
  Cos : Trigonometry  Operator=cos
  Gain : Gain  Gain=-1
  Gain1 : Gain  Gain=-1
  Mux : Mux  Inputs=03
  Mux1 : Mux  Inputs=03
  Product : Product  Inputs=04
  Product1 : Product  Inputs=04
  Product2 : Product  Inputs=04
  Product3 : Product  Inputs=03
  Product4 : Product  Inputs=03
  Product5 : Product  Inputs=03
  Product{6..9} (4 alike) : Product
  Sin : Trigonometry
  " Fax" : Outport
  " Fay" : Outport  Port=2
  " Faz" : Outport  Port=3
  " M_ax" : Outport  Port=4
  M_ay : Outport  Port=5
  " M_az" : Outport  Port=6
  " F_a" : Outport  Port=7
  " M_a" : Outport  Port=8
  wires:
  " cl"/1 -> Product/4
  " b"/1 -> Product2/3, Product/2
  "  S_ref"/1 -> Product3/3, Product4/3, Product5/3, Product2/2, Product1/2, Product/3
  " Q_dyna"/1 -> Product3/2, Product4/2, Product5/2, Product2/1, Product1/3, Product/1
  " cm"/1 -> Product1/4
  " c"/1 -> Product1/1
  " cn"/1 -> Product2/4
  Product1/1 -> Mux/2, M_ay/1
  Product/1 -> Mux/1, " M_ax"/1
  Product2/1 -> Mux/3, " M_az"/1
  CL/1 -> Product5/1
  CD/1 -> Product4/1
  CY/1 -> Product3/1
  Product5/1 -> Product8/1, Product6/2  "L"
  Product4/1 -> Product9/1, Product7/1  "D"
  Product3/1 -> Mux1/2, " Fay"/1  "Fay"
  "  alpha_rad"/1 -> Cos/1, Sin/1
  Sin/1 -> Product9/2, Product6/1
  Cos/1 -> Product7/2, Product8/2
  Product6/1 -> Add/1  "Lsin(a)"
  Product8/1 -> Gain/1  "Lcos(a)"
  Product7/1 -> Add/2  "Dcos(a)"
  Product9/1 -> Gain1/1  "Dsin(a)"
  Gain1/1 -> Add1/2
  Gain/1 -> Add1/1
  Add/1 -> Mux1/1, " Fax"/1
  Mux/1 -> " M_a"/1
  Mux1/1 -> " F_a"/1
  Add1/1 -> " Faz"/1, Mux1/3

== system VTOL_Simulink/Subsystem2/ /Signal Builder ==
  Demux : Demux  Tag=STV Demux  Outputs=1
      settings: DisplayOption=none
  FromWs : FromWorkspace  Tag=STV FromWs  VariableName=tuvar
      SigBuilderData=|
      | common.afterFinalStr = 'Extrapolate'
      | common.sampleTime = 0
      | dataSet.timeRange = [0 400]
      | dataSet.name = 'Group 1'
      | sbobj.Groups.Name = 'Group 1'
      | sbobj.Groups.Signals.Name = 'Signal 2'
      | sbobj.Groups.Signals.XData = [0 10 100 350 400]
      | sbobj.Groups.Signals.YData = [0 1.17e-05 1.53 1.54 1.53]
      | sbobj.Groups.TimeRange = [0 400]
  Signal 2 : Outport  Tag=STV Outport
  wires:
  FromWs/1 -> Demux/1
  Demux/1 -> Signal 2/1

== system VTOL_Simulink/Subsystem2/ /Subsystem1 ==
  Input : Inport
  Add : Sum  Inputs=+-
  Constant : Constant  Value=1000
  Display : Display
  Divide : Product  Inputs=*/
  Scope : Scope
  " Throttle" : Outport
  wires:
  Input/1 -> Display/1, Add/1
  Add/1 -> Divide/1
  Constant/1 -> Divide/2, Add/2
  Divide/1 -> Scope/1, " Throttle"/1

== system VTOL_Simulink/Subsystem2/Subsystem/ Body to LPI ==
  phi : Inport
  theta : Inport  Port=2
  psi : Inport  Port=3
  Display : Display
  Fcn : Fcn  Expr=cos(u(2))*cos(u(3))
  Fcn1 : Fcn  Expr=cos(u(3))*sin(u(1))*sin(u(2))-cos(u(1))*sin(u(3))
  Fcn2 : Fcn  Expr=cos(u(1))*sin(u(2))*cos(u(3))+sin(u(1))*sin(u(3))
  Fcn3 : Fcn  Expr=cos(u(2))*sin(u(3))
  Fcn4 : Fcn  Expr=sin(u(3))*sin(u(1))*sin(u(2))+cos(u(1))*cos(u(3))
  Fcn5 : Fcn  Expr=sin(u(3))*cos(u(1))*sin(u(2))-sin(u(1))*cos(u(3))
  Fcn6 : Fcn  Expr=-sin(u(2))
  Fcn7 : Fcn  Expr=sin(u(1))*cos(u(2))
  Fcn8 : Fcn  Expr=cos(u(1))*cos(u(2))
  Mux : Mux  Inputs=3
  Reshape : Reshape  OutputDimensionality=Customize  OutputDimensions=[3,3]
  Vector Concatenate : Concatenate  NumInputs=09
  C_B_E : Outport
  wires:
  Fcn1/1 -> Vector Concatenate/2
  Fcn4/1 -> Vector Concatenate/5
  Mux/1 -> Fcn8/1, Fcn7/1, Fcn6/1, Fcn5/1, Fcn4/1, Fcn3/1, Fcn2/1, Fcn1/1, Fcn/1
  theta/1 -> Mux/2
  Fcn8/1 -> Vector Concatenate/9
  Fcn6/1 -> Vector Concatenate/7
  Fcn5/1 -> Vector Concatenate/6
  Fcn2/1 -> Vector Concatenate/3
  Fcn/1 -> Vector Concatenate/1
  Fcn3/1 -> Vector Concatenate/4
  Fcn7/1 -> Vector Concatenate/8
  phi/1 -> Mux/1
  psi/1 -> Mux/3
  Vector Concatenate/1 -> Reshape/1
  Reshape/1 -> C_B_E/1, Display/1

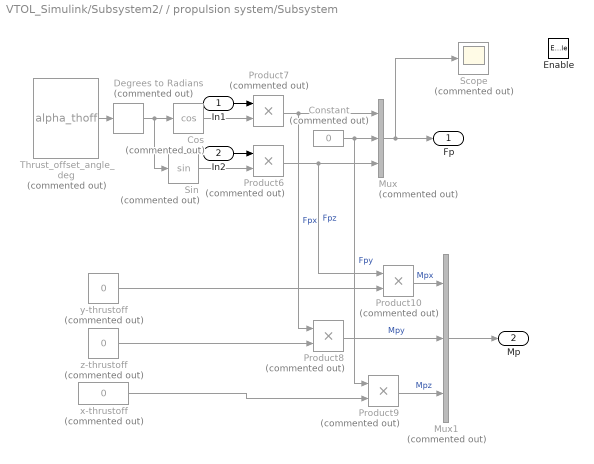
== system VTOL_Simulink/Subsystem2/ / propulsion system/Subsystem ==
  In1 : Inport
  In2 : Inport  Port=2
  Enable : EnablePort
  " Thrust_offset_angle_deg" : Constant  Commented=on  Value=alpha_thoff
  " x-thrustoff" : Constant  Commented=on  Value=0
  " y-thrustoff" : Constant  Commented=on  Value=0
  " z-thrustoff" : Constant  Commented=on  Value=0
  Constant : Constant  Commented=on  Value=0
  Cos : Trigonometry  Commented=on  Operator=cos
  Degrees to Radians : simulink_extras/Transformations/Degrees to Radians  Commented=on
  Mux : Mux  Commented=on  Inputs=03
  Mux1 : Mux  Commented=on  Inputs=03
  Product{6..10} (5 alike) : Product  Commented=on
  Scope : Scope  Commented=on
  Sin : Trigonometry  Commented=on
  " Fp" : Outport
  " Mp" : Outport  Port=2
  wires:
  " z-thrustoff"/1 -> Product8/2
  Product8/1 -> Mux1/2  "Mpy"
  Cos/1 -> Product7/2
  Degrees to Radians/1 -> Sin/1, Cos/1
  In2/1 -> Product6/1
  Mux1/1 -> " Mp"/1
  Constant/1 -> Product9/1, Mux/2  "Fpy"
  In1/1 -> Product7/1
  Product9/1 -> Mux1/3  "Mpz"
  " y-thrustoff"/1 -> Product10/2
  Mux/1 -> " Fp"/1, Scope/1
  Product7/1 -> Product8/1, Mux/1  "Fpx"
  Sin/1 -> Product6/2
  " x-thrustoff"/1 -> Product9/2
  Product10/1 -> Mux1/1  "Mpx"
  Product6/1 -> Product10/1, Mux/3  "Fpz"
  " Thrust_offset_angle_deg"/1 -> Degrees to Radians/1

== matlab function VTOL_Simulink/Subsystem2/ /Tilt angle ==
  data: u input; y output
% function y = fcn(u)
% if (u<=3)
%     y=0;
% elseif(u>3 && u<=15)
%      y=pi*u/30  
% else 
%     y=0; 
% end



function y = fcn(u)
if (u<=3)
    y=0;
elseif(u>3 && u<=15)
     y=pi*u/18-(pi/3);  
else 
    y=pi/2; 
end

== matlab function VTOL_Simulink/Subsystem2/ /MATLAB FuTilt angle ==
  data: t input; y output
function y = fcn(t)
if(t>=0 && t<10)
  y=0;
elseif (t>=10 && t<=20)
  y=(pi/20)*t-pi/2;
else 
   y=pi/2;
end
end

== matlab function VTOL_Simulink/Guidance Mode (u,h,heading Command)/MATLAB Function ==
  data: y output; t input
function y = fcn(t)
 if (t<=10)
    y=-2*t;
 elseif(t>10 && t<=100)
     y=-20;
 elseif(t>100 && t<=140)
     y=t-140;
 else
    y=0;
 end

== matlab function VTOL_Simulink/Guidance Mode (u,h,heading Command)/MATLAB Function3 ==
  data: omega_t output; t input
function omega_t  = fcn(t)
 if(t>500&&t<=550)
     omega_t=1*0.01633;
 else
      omega_t=0; 
 end
